simulink model "AMCLIB_CurrentLoop_BAM"  (Simulink 9.3)
settings: Solver=VariableStepAuto  StartTime=0.0  StopTime=10.0  RelTol=1e-3
settings Model: Creator=nxa18952  LastModifiedBy=nxa18952
settings DataIOCC: SaveFormat=Dataset  SignalLoggingSaveFormat=Dataset  ReturnWorkspaceOutputs=on
settings OptimizationCC: LifeSpan=auto
settings DebuggingCC: UnderspecifiedInitializationDetection=Simplified  MergeDetectMultiDrivingBlocksExec=error  FcnCallInpInsideContextMsg=error  SFUnexpectedBacktrackingDiag=error  SFNoUnconditionalDefaultTransitionDiag=error  SFExecutionAtInitializationDiag=warning  ArithmeticOperatorsInVariantConditions=error
settings HardwareCC: ProdBitPerPointer=64  ProdBitPerSizeT=64  ProdBitPerPtrDiffT=64  ProdLargestAtomicFloat=Float  ProdIntDivRoundTo=Zero  ProdEndianess=LittleEndian  ProdWordSize=64  ProdHWDeviceType=Intel->x86-64 (Windows64)
settings ModelReferenceCC: PropagateSignalLabelsOutOfModel=on
settings SFSimCC: SimUseLocalCustomCode=on
settings RTWCC: RTWUseLocalCustomCode=on
settings CodeAppCC: StateflowObjectComments=off
settings GRTTargetCC: TargetLangStandard=C99 (ISO)  CombineOutputUpdateFcns=on  GRTInterface=off
settings ConfigComp: CovMetricSettings=dwe  CovHtmlReporting=off  CovSaveCumulativeToWorkspaceVar=off  CovSaveSingleToWorkspaceVar=off  CovExternalEMLEnable=on

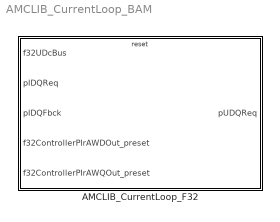
== system AMCLIB_CurrentLoop_BAM ==
  AMCLIB_CurrentLoop_F32 : Subsystem  TreatAsAtomicUnit=on  mask(AMCLIB_CurrentLoop_F32){showStates=Hide (faster execution), resetStatesEnable=Pre-set according to the first set of inputs after reset, f32CC1sc_D=0, f32CC2sc_D=0, u16NShift_D=0, f32CC1sc_Q=0, f32CC2sc_Q=0, u16NShift_Q=0}
      mask prompts: showStates "Show internal states"; resetStatesEnable "Internal state after reset"; f32CC1sc_D "f32CC1sc_D (CC1 coefficient of the D-axis PI controller)"; f32CC2sc_D "f32CC2sc_D (CC2 coefficient of the D-axis PI controller)"; u16NShift_D "u16NShift_D (Scaling bitwise shift applied to the D-axis controller coefficients)"; f32CC1sc_Q "f32CC1sc_Q (CC1 coefficient of the Q-axis PI controller)"; f32CC2sc_Q "f32CC2sc_Q (CC2 coefficient of the Q-axis PI controller)"; u16NShift_Q "u16NShift_Q (Scaling bitwise shift applied to the Q-axis controller coefficients)"
      mask help: Current control loop of the PMSM field-oriented control algorithm in 32-bit fixed-point fractional implementation. This block supports re-initialization of the internal state during simulation. If the block is reset, the outputs of the PI controllers will be aligned with the inputs f32ControllerPIrAWDOut_preset and f32ControllerPIrAWQOut_preset. Refer to the AMMCLIB User's Guide for further details.
      mask init:
      | if ~evalin('base','exist(''tS8'',''var'')')
      |   if (2 ~= exist('SWLIBS_Typedefs.mat','file'))
      |       error('File SWLIBS_Typedefs.mat is not on the Matlab path. Please add the AMMCLIB "bam" folder in the Matlab Search Path.');
      |   else
      |       evalin('base', 'load(''SWLIBS_Typedefs.mat'')');
      |   end
      | end
      | if showStates == 1
      |     % hidden state variables
      |     if strcmp(get_param([gcb '/f32CC1sc_D'], 'BlockType'), 'Inport')
      |         posblk = get_param(gcb, 'Position');
      | 
      |         pos = get_param(    [gcb, '/f32CC1sc_D'], 'Position');
      |         orient = get_param( [gcb, '/f32CC1sc_D'], 'Orientation');
      |         delete_block(       [gcb, '/f32CC1sc_D']);
      |         add_block('built-in/Ground', [gcb, '/f32CC1sc_D'], 'Position', pos, 'Orientation', orient);
      | 
      |         pos = get_param(    [gcb, '/f32CC2sc_D'], 'Position');
      |         orient = get_param( [gcb, '/f32CC2sc_D'], 'Orientation');
      |         delete_block(       [gcb, '/f32CC2sc_D']);
      |         add_block('built-in/Ground', [gcb, '/f32CC2sc_D'], 'Position', pos, 'Orientation', orient);
      | 
      |         pos = get_param(    [gcb, '/u16NShift_D'], 'Position');
      |         orient = get_param( [gcb, '/u16NShift_D'], 'Orientation');
      |         delete_block(       [gcb, '/u16NShift_D']);
      |         add_block('built-in/Ground', [gcb, '/u16NShift_D'], 'Position', pos, 'Orientation', orient);
      | 
      |         pos = get_param(    [gcb, '/f32CC1sc_Q'], 'Position');
      |         orient = get_param( [gcb, '/f32CC1sc_Q'], 'Orientation');
      |         delete_block(       [gcb, '/f32CC1sc_Q']);
      |         add_block('built-in/Ground', [gcb, '/f32CC1sc_Q'], 'Position', pos, 'Orientation', orient);
      | 
      |         pos = get_param(    [gcb, '/f32CC2sc_Q'], 'Position');
      |         orient = get_param( [gcb, '/f32CC2sc_Q'], 'Orientation');
      |         delete_block(       [gcb, '/f32CC2sc_Q']);
      |         add_block('built-in/Ground', [gcb, '/f32CC2sc_Q'], 'Position', pos, 'Orientation', orient);
      | 
      |         pos = get_param(    [gcb, '/u16NShift_Q'], 'Position');
      |         orient = get_param( [gcb, '/u16NShift_Q'], 'Orientation');
      |         delete_block(       [gcb, '/u16NShift_Q']);
      |         add_block('built-in/Ground', [gcb, '/u16NShift_Q'], 'Position', pos, 'Orientation', orient);
      | 
      |         pos = get_param(    [gcb, '/f32Acc_D'], 'Position');
      |         orient = get_param( [gcb, '/f32Acc_D'], 'Orientation');
      |         delete_block(       [gcb, '/f32Acc_D']);
      |         add_block('built-in/Ground', [gcb, '/f32Acc_D'], 'Position', pos, 'Orientation', orient);
      | 
      |         pos = get_param(    [gcb, '/f32InErrK1_D'], 'Position');
      |         orient = get_param( [gcb, '/f32InErrK1_D'], 'Orientation');
      |         delete_block(       [gcb, '/f32InErrK1_D']);
      |         add_block('built-in/Ground', [gcb, '/f32InErrK1_D'], 'Position', pos, 'Orientation', orient);
      | 
      |         pos = get_param(    [gcb, '/f32Acc_Q'], 'Position');
      |         orient = get_param( [gcb, '/f32Acc_Q'], 'Orientation');
      |         delete_block(       [gcb, '/f32Acc_Q']);
      |         add_block('built-in/Ground', [gcb, '/f32Acc_Q'], 'Position', pos, 'Orientation', orient);
      | 
      |         pos = get_param(    [gcb, '/f32InErrK1_Q'], 'Position');
      |         orient = get_param( [gcb, '/f32InErrK1_Q'], 'Orientation');
      |         delete_block(       [gcb, '/f32InErrK1_Q']);
      |         add_block('built-in/Ground', [gcb, '/f32InErrK1_Q'], 'Position', pos, 'Orientation', orient);
      | 
      | 
      |         pos = get_param(    [gcb '/f32Acc_D_Out'], 'Position');
      |         orient = get_param( [gcb '/f32Acc_D_Out'], 'Orientation');
      |         delete_block(       [gcb '/f32Acc_D_Out']);
      |         add_block('built-in/Terminator', [gcb '/f32Acc_D_Out'], 'Position', pos, 'Orientation', orient);
      | 
      |         pos = get_param(    [gcb '/f32InErrK1_D_Out'], 'Position');
      |         orient = get_param( [gcb '/f32InErrK1_D_Out'], 'Orientation');
      |         delete_block(       [gcb '/f32InErrK1_D_Out']);
      |         add_block('built-in/Terminator', [gcb '/f32InErrK1_D_Out'], 'Position', pos, 'Orientation', orient);
      | 
      |         pos = get_param(    [gcb '/f32Acc_Q_Out'], 'Position');
      |         orient = get_param( [gcb '/f32Acc_Q_Out'], 'Orientation');
      |         delete_block(       [gcb '/f32Acc_Q_Out']);
      |         add_block('built-in/Terminator', [gcb '/f32Acc_Q_Out'], 'Position', pos, 'Orientation', orient);
      | 
      |         pos = get_param(    [gcb '/f32InErrK1_Q_Out'], 'Position');
      |         orient = get_param( [gcb '/f32InErrK1_Q_Out'], 'Orientation');
      |         delete_block(       [gcb '/f32InErrK1_Q_Out']);
      |         add_block('built-in/Terminator', [gcb '/f32InErrK1_Q_Out'], 'Position', pos, 'Orientation', orient);
      | 
      | 
      |         set_param([gcb '/f32UDcBus'], 'Port', '1');
      |         set_param([gcb '/pIDQReq'], 'Port', '2');
      |         set_param([gcb '/pIDQFbck'], 'Port', '3');
      |         set_param([gcb '/f32ControllerPIrAWDOut_preset'], 'Port', '4');
      |         set_param([gcb '/f32ControllerPIrAWQOut_preset'], 'Port', '5');
      | 
      |         set_param([gcb '/pUDQReq'], 'Port', '1');
      | 
      |         set_param(gcb,'MaskEnables',{'on','on','on','on','on','on','on','on'});
      | 
      |         if (posblk(4) - posblk(2)) > 150
      |           height = 150;
      |           set_param(gcb,'Position',[posblk(1), posblk(2), posblk(3), posblk(2)+height])
      |         end
      |     end
      | else
      |     % shown state variables
      |     if strcmp(get_param([gcb '/f32CC1sc_D'], 'BlockType'), 'Ground')
      |         posblk = get_param(gcb, 'Position');
      | 
      |         pos = get_param(    [gcb, '/f32CC1sc_D'], 'Position');
      |         orient = get_param( [gcb, '/f32CC1sc_D'], 'Orientation');
      |         delete_block(       [gcb, '/f32CC1sc_D']);
      |         add_block('built-in/Inport', [gcb, '/f32CC1sc_D'], 'Position', pos, 'Orientation', orient, 'OutDataTypeStr', 'int32');
      | 
      |         pos = get_param(    [gcb, '/f32CC2sc_D'], 'Position');
      |         orient = get_param( [gcb, '/f32CC2sc_D'], 'Orientation');
      |         delete_block(       [gcb, '/f32CC2sc_D']);
      |         add_block('built-in/Inport', [gcb, '/f32CC2sc_D'], 'Position', pos, 'Orientation', orient, 'OutDataTypeStr', 'int32');
      | 
      |         pos = get_param(    [gcb, '/u16NShift_D'], 'Position');
      |         orient = get_param( [gcb, '/u16NShift_D'], 'Orientation');
      |         delete_block(       [gcb, '/u16NShift_D']);
      |         add_block('built-in/Inport', [gcb, '/u16NShift_D'], 'Position', pos, 'Orientation', orient, 'OutDataTypeStr', 'uint16');
      | 
      |         pos = get_param(    [gcb, '/f32CC1sc_Q'], 'Position');
      |         orient = get_param( [gcb, '/f32CC1sc_Q'], 'Orientation');
      |         delete_block(       [gcb, '/f32CC1sc_Q']);
      |         add_block('built-in/Inport', [gcb, '/f32CC1sc_Q'], 'Position', pos, 'Orientation', orient, 'OutDataTypeStr', 'int32');
      | 
      |         pos = get_param(    [gcb, '/f32CC2sc_Q'], 'Position');
      |         orient = get_param( [gcb, '/f32CC2sc_Q'], 'Orientation');
      |         delete_block(       [gcb, '/f32CC2sc_Q']);
      |         add_block('built-in/Inport', [gcb, '/f32CC2sc_Q'], 'Position', pos, 'Orientation', orient, 'OutDataTypeStr', 'int32');
      | 
      |         pos = get_param(    [gcb, '/u16NShift_Q'], 'Position');
      |         orient = get_param( [gcb, '/u16NShift_Q'], 'Orientation');
      |         delete_block(       [gcb, '/u16NShift_Q']);
      |         add_block('built-in/Inport', [gcb, '/u16NShift_Q'], 'Position', pos, 'Orientation', orient, 'OutDataTypeStr', 'uint16');
      | 
      |         pos = get_param(    [gcb, '/f32Acc_D'], 'Position');
      |         orient = get_param( [gcb, '/f32Acc_D'], 'Orientation');
      |         delete_block(       [gcb, '/f32Acc_D']);
      |         add_block('built-in/Inport', [gcb, '/f32Acc_D'], 'Position', pos, 'Orientation', orient, 'OutDataTypeStr', 'int32');
      | 
      |         pos = get_param(    [gcb, '/f32InErrK1_D'], 'Position');
      |         orient = get_param( [gcb, '/f32InErrK1_D'], 'Orientation');
      |         delete_block(       [gcb, '/f32InErrK1_D']);
      |         add_block('built-in/Inport', [gcb, '/f32InErrK1_D'], 'Position', pos, 'Orientation', orient, 'OutDataTypeStr', 'int32');
      | 
      |         pos = get_param(    [gcb, '/f32Acc_Q'], 'Position');
      |         orient = get_param( [gcb, '/f32Acc_Q'], 'Orientation');
      |         delete_block(       [gcb, '/f32Acc_Q']);
      |         add_block('built-in/Inport', [gcb, '/f32Acc_Q'], 'Position', pos, 'Orientation', orient, 'OutDataTypeStr', 'int32');
      | 
      |         pos = get_param(    [gcb, '/f32InErrK1_Q'], 'Position');
      |         orient = get_param( [gcb, '/f32InErrK1_Q'], 'Orientation');
      |         delete_block(       [gcb, '/f32InErrK1_Q']);
      |         add_block('built-in/Inport', [gcb, '/f32InErrK1_Q'], 'Position', pos, 'Orientation', orient, 'OutDataTypeStr', 'int32');
      | 
      | 
      |         pos = get_param(    [gcb '/f32Acc_D_Out'], 'Position');
      |         orient = get_param( [gcb '/f32Acc_D_Out'], 'Orientation');
      |         delete_block(       [gcb '/f32Acc_D_Out']);
      |         add_block('built-in/Outport', [gcb '/f32Acc_D_Out'], 'Position', pos, 'Orientation', orient);
      | 
      |         pos = get_param(    [gcb '/f32InErrK1_D_Out'], 'Position');
      |         orient = get_param( [gcb '/f32InErrK1_D_Out'], 'Orientation');
      |         delete_block(       [gcb '/f32InErrK1_D_Out']);
      |         add_block('built-in/Outport', [gcb '/f32InErrK1_D_Out'], 'Position', pos, 'Orientation', orient);
      | 
      |         pos = get_param(    [gcb '/f32Acc_Q_Out'], 'Position');
      |         orient = get_param( [gcb '/f32Acc_Q_Out'], 'Orientation');
      |         delete_block(       [gcb '/f32Acc_Q_Out']);
      |         add_block('built-in/Outport', [gcb '/f32Acc_Q_Out'], 'Position', pos, 'Orientation', orient);
      | 
      |         pos = get_param(    [gcb '/f32InErrK1_Q_Out'], 'Position');
      |         orient = get_param( [gcb '/f32InErrK1_Q_Out'], 'Orientation');
      |         delete_block(       [gcb '/f32InErrK1_Q_Out']);
      |         add_block('built-in/Outport', [gcb '/f32InErrK1_Q_Out'], 'Position', pos, 'Orientation', orient);
      | 
      | 
      |         set_param([gcb '/f32UDcBus'], 'Port', '1');
      |         set_param([gcb '/pIDQReq'], 'Port', '2');
      |         set_param([gcb '/pIDQFbck'], 'Port', '3');
      |         set_param([gcb '/f32ControllerPIrAWDOut_preset'], 'Port', '4');
      |         set_param([gcb '/f32ControllerPIrAWQOut_preset'], 'Port', '5');
      |         set_param([gcb '/f32CC1sc_D'], 'Port', '6');
      |         set_param([gcb '/f32CC2sc_D'], 'Port', '7');
      |         set_param([gcb '/u16NShift_D'], 'Port', '8');
      |         set_param([gcb '/f32CC1sc_Q'], 'Port', '9');
      |         set_param([gcb '/f32CC2sc_Q'], 'Port', '10');
      |         set_param([gcb '/u16NShift_Q'], 'Port', '11');
      |         set_param([gcb '/f32Acc_D'], 'Port', '12');
      |         set_param([gcb '/f32InErrK1_D'], 'Port', '13');
      |         set_param([gcb '/f32Acc_Q'], 'Port', '14');
      |         set_param([gcb '/f32InErrK1_Q'], 'Port', '15');
      | 
      |         set_param([gcb '/pUDQReq'], 'Port', '1');
      |         set_param([gcb '/f32Acc_D_Out'], 'Port', '2');
      |         set_param([gcb '/f32InErrK1_D_Out'], 'Port', '3');
      |         set_param([gcb '/f32Acc_Q_Out'], 'Port', '4');
      |         set_param([gcb '/f32InErrK1_Q_Out'], 'Port', '5');
      | 
      |         set_param(gcb,'MaskEnables',{'on','on','off','off','off','off','off','off'});
      | 
      |         if (posblk(4) - posblk(2)) < 400
      |           height = 400;
      |           set_param(gcb,'Position',[posblk(1), posblk(2), posblk(3), posblk(2)+height])
      |         end
      |     end
      | end
      settings: RTWSystemCode=Inline
      mask TypeOptions showStates: Hide (faster execution) | Show (allows debugging; connect feedback loops manually)
      mask Callback showStates:
      | maskStr = get_param(gcb,'showStates');
      | if strcmp(maskStr,'Hide (faster execution)'),
      |     set_param(gcb,'MaskEnables',{'on','on','on','on','on','on','on','on'});
      | else
      |     set_param(gcb,'MaskEnables',{'on','on','off','off','off','off','off','off'});
      | end
      mask TypeOptions resetStatesEnable: Pre-set according to the first set of inputs after reset | Clear to zero
      mask Display:
      | color('black');
      | pos = get_param(gcb, 'Position');
      | width = pos(3) - pos(1);
      | height = pos(4) - pos(2);
      | tX=width/2;
      | tY=height - 25;
      | color('black');
      | text(tX,tY, 'AMCLIB_CurrentLoop_F32', 'horizontalAlignment', 'center');
      | if showStates == 2
      |   color('red');
      |   text(tX,tY - 20, ['debugging mode' char(13) char(10) '(limited performance)'], 'horizontalAlignment', 'center');
      | end

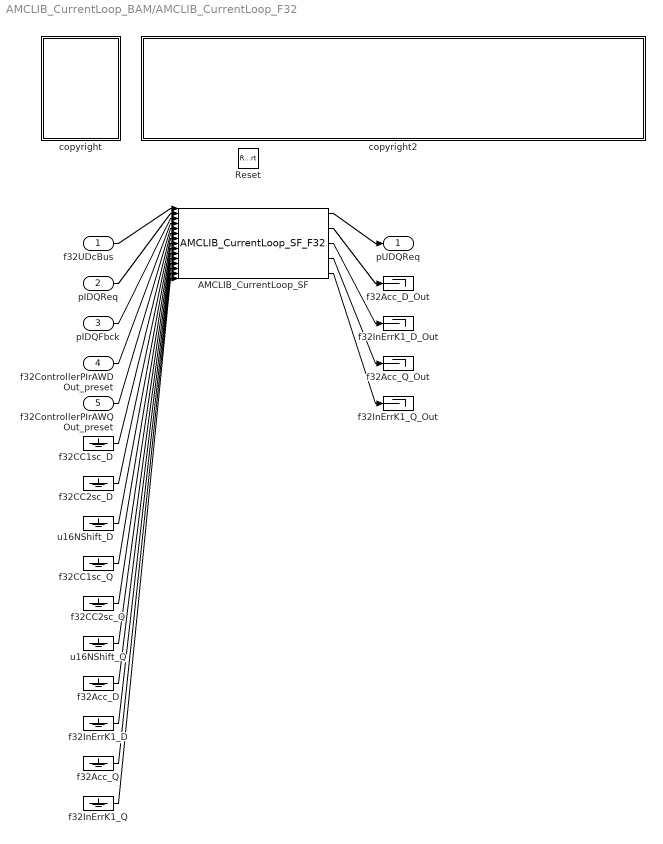
== system AMCLIB_CurrentLoop_BAM/AMCLIB_CurrentLoop_F32 ==
  f32UDcBus : Inport  OutDataTypeStr=int32
  pIDQReq : Inport  Port=2  OutDataTypeStr=Bus: SWLIBS_2Syst_F32  BusOutputAsStruct=on
  pIDQFbck : Inport  Port=3  OutDataTypeStr=Bus: SWLIBS_2Syst_F32  BusOutputAsStruct=on
  f32ControllerPIrAWDOut_preset : Inport  Port=4  OutDataTypeStr=int32
  f32ControllerPIrAWQOut_preset : Inport  Port=5  OutDataTypeStr=int32
  Reset : ResetPort  DisableCoverage=on
  AMCLIB_CurrentLoop_SF : S-Function  FunctionName=AMCLIB_CurrentLoop_SF_F32  Parameters=showStates,resetStatesEnable,f32CC1sc_D,f32CC2sc_D,u16NShift_D,f32CC1sc_Q,f32CC2sc_Q,u16NShift_Q  SFunctionDeploymentMode=off  EnableBusSupport=off
  copyright : Subsystem
      mask Display: text(10,90,'FILE:');text(10,75,'DESRIPTION:');text(10,60,'COPYRIGHT:');text(10,45,'VERSION:');text(10,30,'DATE:')
  copyright2 : Subsystem
      mask Display: text(10,90,'AMCLIB_CurrentLoop_BAM_F32.mdl');text(10,75,'PMSM Current Loop.');text(10,60,'NXP 2020');text(10,45,'1.0');text(10,30,'28-Mar-2020');
  f32Acc_D : Ground
  f32Acc_D_Out : Terminator
  f32Acc_Q : Ground
  f32Acc_Q_Out : Terminator
  f32CC1sc_D : Ground
  f32CC1sc_Q : Ground
  f32CC2sc_D : Ground
  f32CC2sc_Q : Ground
  f32InErrK1_D : Ground
  f32InErrK1_D_Out : Terminator
  f32InErrK1_Q : Ground
  f32InErrK1_Q_Out : Terminator
  u16NShift_D : Ground
  u16NShift_Q : Ground
  pUDQReq : Outport
  wires:
  f32UDcBus/1 -> AMCLIB_CurrentLoop_SF/1
  pIDQReq/1 -> AMCLIB_CurrentLoop_SF/2
  pIDQFbck/1 -> AMCLIB_CurrentLoop_SF/3
  f32ControllerPIrAWDOut_preset/1 -> AMCLIB_CurrentLoop_SF/4
  f32ControllerPIrAWQOut_preset/1 -> AMCLIB_CurrentLoop_SF/5
  f32CC1sc_D/1 -> AMCLIB_CurrentLoop_SF/6
  f32CC2sc_D/1 -> AMCLIB_CurrentLoop_SF/7
  u16NShift_D/1 -> AMCLIB_CurrentLoop_SF/8
  f32CC1sc_Q/1 -> AMCLIB_CurrentLoop_SF/9
  f32CC2sc_Q/1 -> AMCLIB_CurrentLoop_SF/10
  u16NShift_Q/1 -> AMCLIB_CurrentLoop_SF/11
  f32Acc_D/1 -> AMCLIB_CurrentLoop_SF/12
  f32InErrK1_D/1 -> AMCLIB_CurrentLoop_SF/13
  f32Acc_Q/1 -> AMCLIB_CurrentLoop_SF/14
  f32InErrK1_Q/1 -> AMCLIB_CurrentLoop_SF/15
  AMCLIB_CurrentLoop_SF/1 -> pUDQReq/1
  AMCLIB_CurrentLoop_SF/2 -> f32Acc_D_Out/1
  AMCLIB_CurrentLoop_SF/3 -> f32InErrK1_D_Out/1
  AMCLIB_CurrentLoop_SF/4 -> f32Acc_Q_Out/1
  AMCLIB_CurrentLoop_SF/5 -> f32InErrK1_Q_Out/1

== system AMCLIB_CurrentLoop_BAM/AMCLIB_CurrentLoop_F32/copyright ==

== system AMCLIB_CurrentLoop_BAM/AMCLIB_CurrentLoop_F32/copyright2 ==
